simulink model "adder_single"  (R2023b)
settings: Solver=VariableStepAuto  StartTime=0.0  StopTime=inf  RelTol=1e-3
libraries: simulink x2
settings Model: Creator=yk  LastModifiedBy=cqupt-Guoping
settings OptimizationCC: BlockReduction=off  ConditionallyExecuteInputs=off  DefaultParameterBehavior=Inlined
settings DebuggingCC: AlgebraicLoopMsg=error
settings HardwareCC: ProdBitPerPointer=32  ProdBitPerSizeT=32  ProdBitPerPtrDiffT=32  ProdLargestAtomicFloat=None  ProdIntDivRoundTo=Undefined  ProdEndianess=Unspecified  ProdWordSize=32  ProdHWDeviceType=ASIC/FPGA->ASIC/FPGA  TargetBitPerPointer=64  TargetBitPerSizeT=64  TargetBitPerPtrDiffT=64  TargetLongLongMode=on  TargetIntDivRoundTo=Zero  TargetEndianess=LittleEndian  TargetWordSize=64  TargetHWDeviceType=Custom Processor->MATLAB Host Computer  ProdEqTarget=off

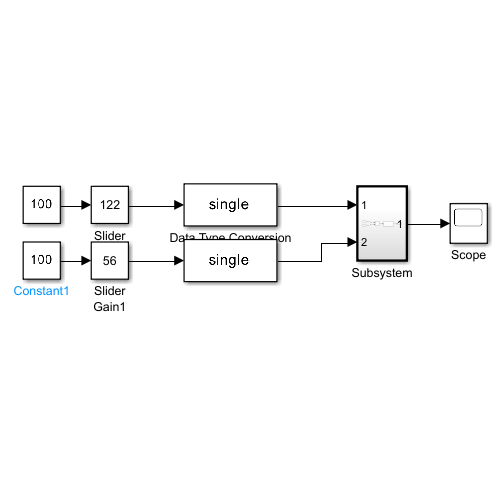
[thumbnail: Simulink's stored preview of the top-level diagram]
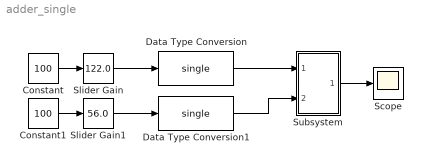
== system adder_single ==
  Constant : Constant  Value=100
  Constant1 : Constant  Value=100
  Data Type Conversion : DataTypeConversion  OutDataTypeStr=single  SaturateOnIntegerOverflow=off  RndMeth=Floor
  Data Type Conversion1 : DataTypeConversion  OutDataTypeStr=single  SaturateOnIntegerOverflow=off  RndMeth=Floor
  Scope : Scope
  Slider Gain : simulink/Math Operations/Slider Gain  gain=122.0  low=0  high=200
  Slider Gain1 : simulink/Math Operations/Slider Gain  gain=56.0  low=0  high=200
  Subsystem : Subsystem  TreatAsAtomicUnit=on
  wires:
  Subsystem/1(Out1) -> Scope/1
  Constant/1 -> Slider Gain/1
  Constant1/1 -> Slider Gain1/1
  Slider Gain/1 -> Data Type Conversion/1
  Data Type Conversion/1 -> Subsystem/1(In1)
  Slider Gain1/1 -> Data Type Conversion1/1
  Data Type Conversion1/1 -> Subsystem/2(In2)

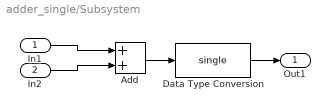
== system adder_single/Subsystem ==
  In1 : Inport  OutDataTypeStr=single  SampleTime=10e-9
  In2 : Inport  Port=2  OutDataTypeStr=single  SampleTime=10e-9
  Add : Sum
  Data Type Conversion : DataTypeConversion  OutDataTypeStr=single  SaturateOnIntegerOverflow=off  RndMeth=Floor
  Out1 : Outport  OutDataTypeStr=single
  wires:
  In2/1 -> Add/2
  In1/1 -> Add/1
  Add/1 -> Data Type Conversion/1
  Data Type Conversion/1 -> Out1/1
